simulink subsystem "MPC12_nlpsol"  (R2022b)
settings: Solver=VariableStepAuto  StartTime=0.0  StopTime=10.0  RelTol=1e-3
undefined symbols (not defined in the file): param_jointspace_ct, param_MPC12, param_robot, param_traj, param_weight_init
settings Model: Creator=emu  LastModifiedBy=emu
settings OptimizationCC: ReuseModelBlockBuffer=on

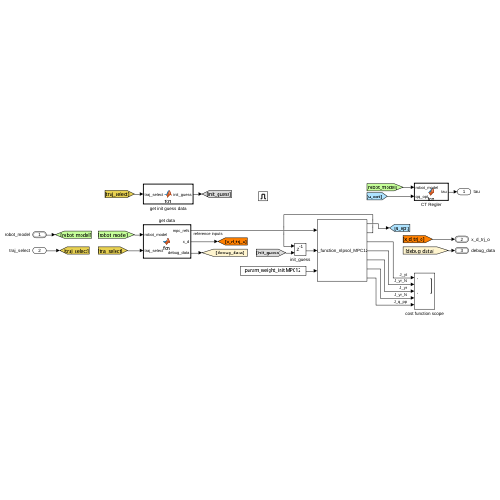
[thumbnail: Simulink's stored preview of the top-level diagram]
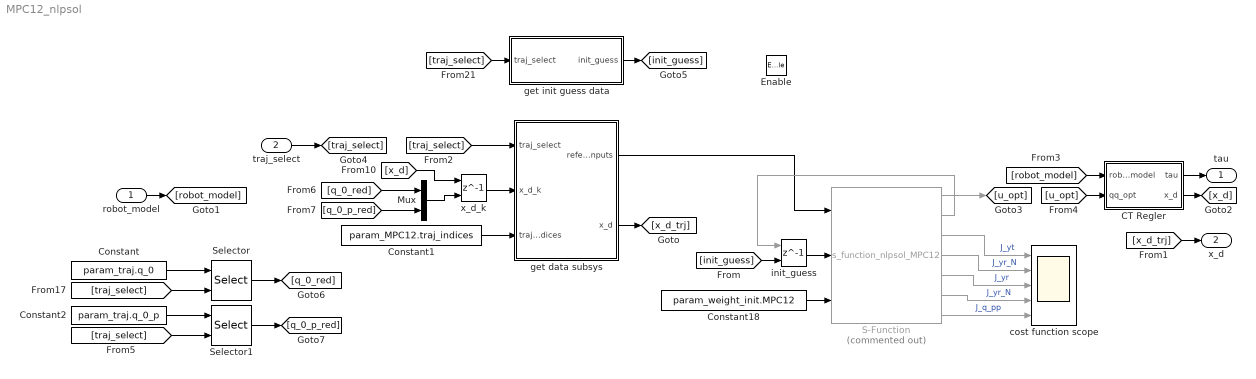
== system MPC12_nlpsol ==
  robot_model : Inport  OutDataTypeStr=Bus: robot_model
  traj_select : Inport  Port=2
  Enable : EnablePort
  CT Regler : MATLAB Function  TreatAsAtomicUnit=on
  Constant : Constant  Value=param_traj.q_0
  Constant1 : Constant  Value=param_MPC12.traj_indices
  Constant18 : Constant  Value=param_weight_init.MPC12  VectorParams1D=off
  Constant2 : Constant  Value=param_traj.q_0_p
  Mux : Mux  Inputs=2
  S-Function : S-Function  Commented=on  FunctionName=s_function_nlpsol_MPC12  Parameters='s_functions/fr3_no_hand_6dof/MPC12.casadi', 'MPC12'  SFunctionModules='MPC12'  SFunctionDeploymentMode=off  EnableBusSupport=off
  Selector : Selector  NumberOfDimensions=2  InputPortWidth=3  IndexOptions=Index vector (dialog),Index vector (port)  Indices=param_robot.n_indices,1  OutputSizes=1,1
  Selector1 : Selector  NumberOfDimensions=2  InputPortWidth=3  IndexOptions=Index vector (dialog),Index vector (port)  Indices=param_robot.n_indices,1  OutputSizes=1,1
  cost function scope : Scope  NumInputPorts=5
  get data subsys : Subsystem
  get init guess data : MATLAB Function  TreatAsAtomicUnit=on
  init_guess : Delay  DelayLength=1  InitialConditionSource=Input port  InitialCondition=1
      settings: InputPortMap=u0,p4
  x_d_k : Delay  DelayLength=1  InitialConditionSource=Input port  InitialCondition=1
      settings: InputPortMap=u0,p4
  tau : Outport
  x_d : Outport  Port=2  OutDataTypeStr=Bus: x_d
  wires:
  get data subsys/2(x_d) -> [x_d_trj]
  get data subsys/1(reference inputs) -> S-Function/1
  Constant1/1 -> get data subsys/3(traj_indices)
  x_d_k/1 -> get data subsys/2(x_d_k)
  [traj_select] -> get data subsys/1(traj_select)
  [x_d_trj] -> x_d/1
  Mux/1 -> x_d_k/2
  [q_0_p_red] -> Mux/2
  [q_0_red] -> Mux/1
  CT Regler/2(x_d) -> [x_d]
  [x_d] -> x_d_k/1
  S-Function/1 -> [u_opt]
  S-Function/5 -> cost function scope/3  "J_yr"
  S-Function/3 -> cost function scope/1  "J_yt"
  Constant18/1 -> S-Function/3
  get init guess data/1(init_guess) -> [init_guess]
  init_guess/1 -> S-Function/2
  robot_model/1 -> [robot_model]
  [robot_model] -> CT Regler/1(robot_model)
  S-Function/4 -> cost function scope/2  "J_yr_N"
  [u_opt] -> CT Regler/2(qq_opt)
  traj_select/1 -> [traj_select]
  S-Function/6 -> cost function scope/4  "J_yr_N"
  CT Regler/1(tau) -> tau/1
  [init_guess] -> init_guess/2
  [traj_select] -> get init guess data/1(traj_select)
  S-Function/7 -> cost function scope/5  "J_q_pp"
  S-Function/2 -> init_guess/1
  Constant2/1 -> Selector1/1
  Constant/1 -> Selector/1
  [traj_select] -> Selector/2
  [traj_select] -> Selector1/2
  Selector/1 -> [q_0_red]
  Selector1/1 -> [q_0_p_red]

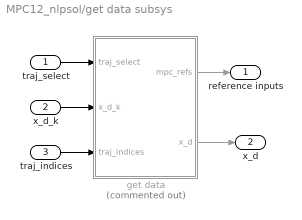
== system MPC12_nlpsol/get data subsys ==
  traj_select : Inport
  x_d_k : Inport  Port=2
  traj_indices : Inport  Port=3
  get data : MATLAB Function  Commented=on  TreatAsAtomicUnit=on
  reference inputs : Outport
  x_d : Outport  Port=2  OutDataTypeStr=Bus: x_d
  wires:
  traj_indices/1 -> get data/3(traj_indices)
  get data/2(x_d) -> x_d/1
  x_d_k/1 -> get data/2(x_d_k)
  get data/1(mpc_refs) -> reference inputs/1
  traj_select/1 -> get data/1(traj_select)

== matlab function MPC12_nlpsol/CT Regler ==
  data: robot_model input Bus: robot_model; tau output; qq_opt input; param_robot parameter; param_jointspace_ct parameter; x_d output
function [tau, x_d] = fcn(robot_model, qq_opt, param_robot, param_jointspace_ct)

n_indices = param_robot.n_indices;

n_red = param_robot.n_red;
q = robot_model.q;      % generalized coordinates
q_p = robot_model.q_p;  % time derivative of generalized coordinates

if size(qq_opt, 2) ~= 0 && size(qq_opt, 1) ~= 1
    q_d_0 = qq_opt(1:n_red, 1); % q_0
    q_d_0_p = qq_opt(n_red+1:2*n_red, 1); %q_p_0
    q_d_0_pp = qq_opt(2*n_red+1:3*n_red, 1); %q_p_00
    
    M_red = robot_model.M(n_indices, n_indices);      % inertia matrix
    C_rnea_red = robot_model.C_rnea(n_indices); % C_rnea(q, q_p) = C(q, q_p)q_p + g(q) = n(q, q_p)
    
    e = q(n_indices) - q_d_0;
    e_p = q_p(n_indices) - q_d_0_p;
    
    K_D_q = param_jointspace_ct.MPC12.K_D_q(n_indices, n_indices);
    K_P_q = param_jointspace_ct.MPC12.K_P_q(n_indices, n_indices);
    tau = M_red*(q_d_0_pp - K_D_q * e_p - K_P_q * e) + C_rnea_red;

    q_d_1 = qq_opt(1+3*n_red:4*n_red, 1); % q_0
    q_d_1_p = qq_opt(1+4*n_red:5*n_red, 1); %q_p_0

    x_d = [q_d_1; q_d_1_p];
else
    tau = zeros(n_red,1);
    x_d = [q(n_indices); q_p(n_indices)];
end

== matlab function MPC12_nlpsol/get data subsys/get data ==
  settings: updateMethod=DISCRETE  sampleTime=param_global.Ta
  data: mpc_refs output; param_traj_data parameter; traj_select input; x_d_k input; traj_indices input; x_d output Bus: x_d
function [mpc_refs, x_d] = fcn(param_traj_data, traj_select, x_d_k, traj_indices)
persistent cnt;

if(isempty(cnt))
    cnt = 1;
end

traj_indices = traj_indices + (cnt-1);

% Parameters
x_k = x_d_k; % open loop mpc

% Assemble vector of recieved output measurements
p_d     = param_traj_data.p_d(   1:3, traj_indices, traj_select);
q_d     = param_traj_data.q_d(   1:4, traj_indices, traj_select);

y_d = [p_d; q_d];

%% Reference out
mpc_refs = [x_k(:); y_d(:)];

%% Offline Trajectory out
x_d.p_d            = param_traj_data.p_d(           :,    cnt, traj_select);
x_d.p_d_p          = param_traj_data.p_d_p(         :,    cnt, traj_select);
x_d.p_d_pp         = param_traj_data.p_d_pp(        :,    cnt, traj_select);
x_d.Phi_d          = param_traj_data.Phi_d(         :,    cnt, traj_select);
x_d.Phi_d_p        = param_traj_data.Phi_d_p(       :,    cnt, traj_select);
x_d.Phi_d_pp       = param_traj_data.Phi_d_pp(      :,    cnt, traj_select);
x_d.R_d            = param_traj_data.R_d(           :, :, cnt, traj_select);
x_d.q_d            = param_traj_data.q_d(           :,    cnt, traj_select);
x_d.q_d_p          = param_traj_data.q_d_p(         :,    cnt, traj_select);
x_d.q_d_pp         = param_traj_data.q_d_pp(        :,    cnt, traj_select);
x_d.omega_d        = param_traj_data.omega_d(       :,    cnt, traj_select);
x_d.omega_d_p      = param_traj_data.omega_d_p(     :,    cnt, traj_select);
x_d.alpha_d        = param_traj_data.alpha_d(       :,    cnt, traj_select);
x_d.alpha_d_p      = param_traj_data.alpha_d_p(     :,    cnt, traj_select);
x_d.alpha_d_pp     = param_traj_data.alpha_d_pp(    :,    cnt, traj_select);
x_d.rot_ax_d       = param_traj_data.rot_ax_d(      :,    cnt, traj_select);
x_d.alpha_d_offset = param_traj_data.alpha_d_offset(:,    cnt, traj_select);
x_d.q_d_rel        = param_traj_data.q_d_rel(       :,    cnt, traj_select);

cnt = cnt+1;

== matlab function MPC12_nlpsol/get init guess data ==
  data: traj_select input; param_MPC12_init_guess parameter; init_guess output
function init_guess   = fcn(traj_select, param_MPC12_init_guess)

init_guess = param_MPC12_init_guess.init_guess(traj_select,:);
